simulink model "maglevAGH"  (R2020a)
settings: Solver=ode45  StartTime=0.0  StopTime=1  MaxStep=0.001  RelTol=1e-3  EnableMultiTasking=on
values from neighbouring files (symbols this model uses):
  g_E = 9.81    [identification_data.m]
  i_ep = sqrt(-2*m_b*g_E/L_d_ep)    [identification_data.m]
  m_b = 58e-3    (= 0.058)    [identification_data.m]
  R_n = mean(R(1:end-1))    [identification_data.m]
  u_ep = R_n * i_ep    [identification_data.m]
undefined symbols (not defined in the file or in its folder): ind
settings Model: Creator=tutaj  LastModifiedBy=wkula
settings DataIOCC: LimitDataPoints=on  SaveFormat=Array  ReturnWorkspaceOutputs=off
settings OptimizationCC: LifeSpan=inf
settings DebuggingCC: UnderspecifiedInitializationDetection=Classic  MergeDetectMultiDrivingBlocksExec=none  SolverPrmCheckMsg=warning  StateNameClashWarn=warning  SFUnexpectedBacktrackingDiag=warning  SFNoUnconditionalDefaultTransitionDiag=warning  SFExecutionAtInitializationDiag=none  ArithmeticOperatorsInVariantConditions=warning
settings HardwareCC: ProdBitPerPointer=32  ProdBitPerSizeT=32  ProdBitPerPtrDiffT=32  ProdLargestAtomicFloat=None  ProdIntDivRoundTo=Undefined  ProdEndianess=Unspecified  ProdWordSize=32  ProdHWDeviceType=32-bit Generic
settings ModelReferenceCC: PropagateSignalLabelsOutOfModel=off
settings SFSimCC: SimUseLocalCustomCode=off  CustomCodeUndefinedFunction=UseInterfaceOnly
settings RTWCC: RTWUseLocalCustomCode=off
settings CodeAppCC: StateflowObjectComments=on
settings GRTTargetCC: TargetLangStandard=C89/C90 (ANSI)
settings ConfigComp: CovMetricSettings=dw  CovHtmlReporting=on  CovSaveCumulativeToWorkspaceVar=on  CovSaveSingleToWorkspaceVar=on  CovExternalEMLEnable=off

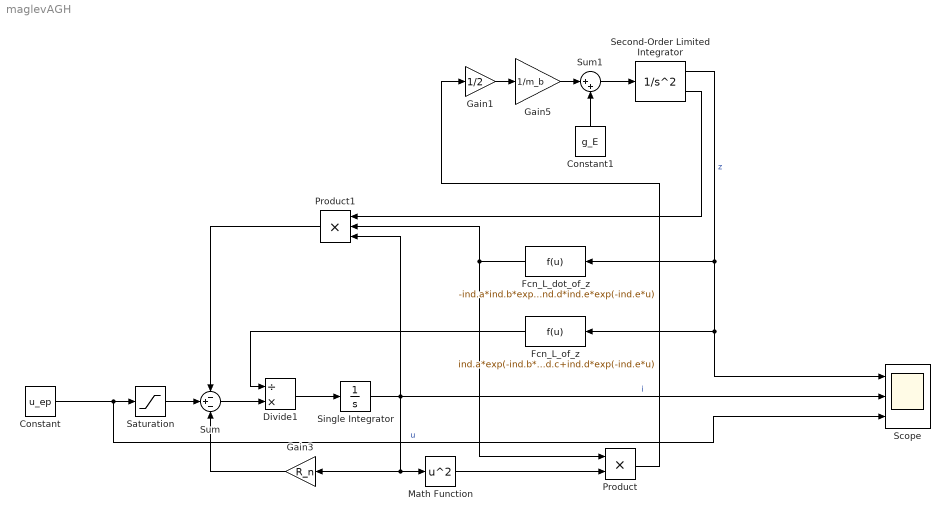
== system maglevAGH ==
  Constant : Constant  Value=u_ep
  Constant1 : Constant  Value=g_E
  Divide1 : Product  Inputs=/*
  Fcn_L_dot_of_z : Fcn  Expr=-ind.a*ind.b*exp(-ind.b*u)-ind.d*ind.e*exp(-ind.e*u)
  Fcn_L_of_z : Fcn  Expr=ind.a*exp(-ind.b*u)+ind.c+ind.d*exp(-ind.e*u)
  Gain1 : Gain  Gain=1/2
  Gain3 : Gain  Gain=R_n
  Gain5 : Gain  Gain=1/m_b
  Math Function : Math  Operator=square  SignedPower=on  SaturateOnIntegerOverflow=on
  Product : Product
  Product1 : Product  Inputs=3
  Saturation : Saturate  UpperLimit=12  LowerLimit=0
  Scope : Scope  NumInputPorts=3
  Second-Order Limited Integrator : SecondOrderIntegrator  ICX=z_ep  LimitX=on  UpperLimitX=0.2  LowerLimitX=0  ICDXDT=v_ep
  Single Integrator : Integrator  InitialCondition=i_ep
  Sum : Sum  Inputs=-+-
  Sum1 : Sum  Inputs=|++
  wires:
  Saturation/1 -> Sum/2
  Constant1/1 -> Sum1/2
  Constant/1 -> Scope/3, Saturation/1  "u"
  Product1/1 -> Sum/1
  Divide1/1 -> Single Integrator/1
  Math Function/1 -> Product/2
  Fcn_L_of_z/1 -> Divide1/1
  Gain1/1 -> Gain5/1
  Gain5/1 -> Sum1/1
  Fcn_L_dot_of_z/1 -> Product1/2, Product/1
  Sum1/1 -> Second-Order Limited Integrator/1
  Sum/1 -> Divide1/2
  Gain3/1 -> Sum/3
  Product/1 -> Gain1/1
  Single Integrator/1 -> Gain3/1, Math Function/1, Scope/2, Product1/3  "i"
  Second-Order Limited Integrator/1 -> Scope/1, Fcn_L_of_z/1, Fcn_L_dot_of_z/1  "z"
  Second-Order Limited Integrator/2 -> Product1/1
